simulink model "Robot_contour"  (R2021a)
settings: Solver=VariableStepAuto  StartTime=0.0  StopTime=10.0  RelTol=1e-3

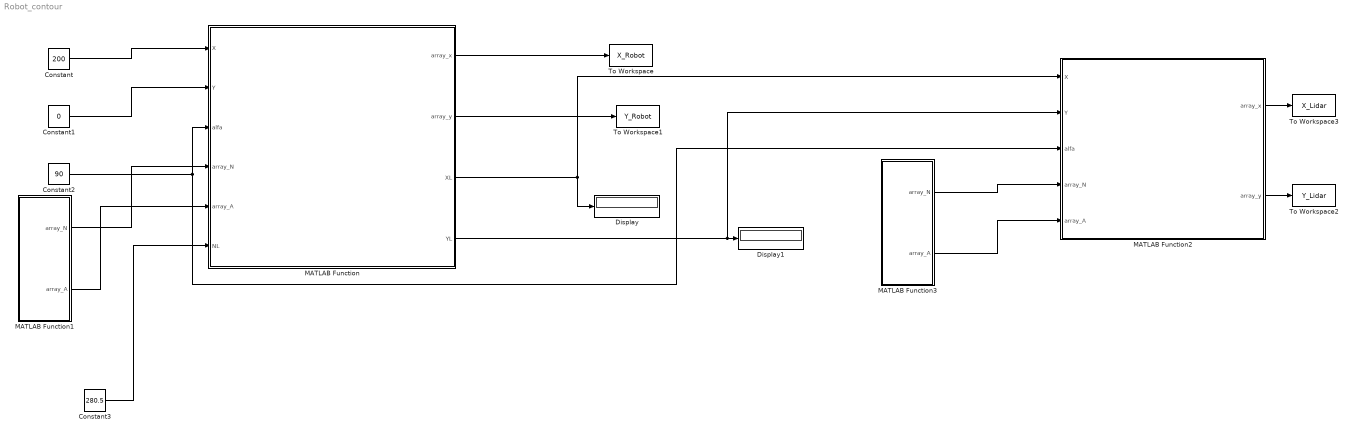
== system Robot_contour ==
  Constant : Constant  Value=200
  Constant1 : Constant  Value=0
  Constant2 : Constant  Value=90
  Constant3 : Constant  Value=280.5
  Display : Display
  Display1 : Display
  MATLAB Function : MATLAB Function  TreatAsAtomicUnit=on
  MATLAB Function1 : MATLAB Function  TreatAsAtomicUnit=on
  MATLAB Function2 : MATLAB Function  TreatAsAtomicUnit=on
  MATLAB Function3 : MATLAB Function  TreatAsAtomicUnit=on
  To Workspace : ToWorkspace  VariableName=X_Robot  SampleTime=10
  To Workspace1 : ToWorkspace  VariableName=Y_Robot  SampleTime=10
  To Workspace2 : ToWorkspace  VariableName=Y_Lidar  SampleTime=10
  To Workspace3 : ToWorkspace  VariableName=X_Lidar  SampleTime=10
  wires:
  MATLAB Function1/1(array_N) -> MATLAB Function/4(array_N)
  MATLAB Function/1(array_x) -> To Workspace/1
  MATLAB Function/2(array_y) -> To Workspace1/1
  MATLAB Function1/2(array_A) -> MATLAB Function/5(array_A)
  Constant3/1 -> MATLAB Function/6(NL)
  MATLAB Function/3(XL) -> MATLAB Function2/1(X), Display/1
  MATLAB Function/4(YL) -> Display1/1, MATLAB Function2/2(Y)
  Constant/1 -> MATLAB Function/1(X)
  Constant1/1 -> MATLAB Function/2(Y)
  Constant2/1 -> MATLAB Function/3(alfa), MATLAB Function2/3(alfa)
  MATLAB Function2/2(array_y) -> To Workspace2/1
  MATLAB Function2/1(array_x) -> To Workspace3/1
  MATLAB Function3/1(array_N) -> MATLAB Function2/4(array_N)
  MATLAB Function3/2(array_A) -> MATLAB Function2/5(array_A)

== matlab function Robot_contour/MATLAB Function3 ==
function [array_N,array_A]=fcn() 

array_N=randi([4000,6000],(360*2),1);
array_A=((0:719)/2);

== matlab function Robot_contour/MATLAB Function1 ==
function [array_N,array_A]=fcn() 

array_N=[367.6,735.29,747.2,390.89,420.92,330.25,648.42,648.42,330.25,420.92,390.89,747.2,735.29,367.6,367.6];
array_A=[9.08,4.52,11.19,21.77,30.41,66.35,152.09,-152.09,-66.35,-30.41,-21.77,-11.19,-4.52,-9.08,9.08];

== matlab function Robot_contour/MATLAB Function ==
function [array_x ,array_y,XL,YL ] = fcn(X,Y,alfa,array_N,array_A,NL)
array_x=zeros(1,15);
array_y=zeros(1,15);
for i=1:15 
array_x(i)= X + array_N(i)*cosd(alfa-array_A(i));
array_y(i)= Y + array_N(i)*sind(alfa-array_A(i));    
end

XL= X + NL*cosd(alfa);
YL= Y + NL*sind(alfa);

== matlab function Robot_contour/MATLAB Function2 ==
function [array_x ,array_y] = fcn(X,Y,alfa,array_N,array_A)
array_x=zeros(1,360*2);
array_y=zeros(1,360*2);
for i=1:(360*2)
array_x(i)= X + array_N(i)*cosd(alfa-array_A(i));
array_y(i)= Y + array_N(i)*sind(alfa-array_A(i));    
end
